simulink model "missile_Lin_model"  (R2022b)
settings: Solver=VariableStepAuto  StartTime=0.0  StopTime=10.0  RelTol=1e-3
InitFcn:
  | UAV_Data
  | Sim_Parameters
values from neighbouring files (symbols this model uses):
  D = 0.150    (= 0.15)    [UAV_Data.m]    (also in UAV_Data.mat)
  I_TENSOR = [ I_xx,  0.0,  0.0 ... (first row only)    [UAV_Data.m]    (also in UAV_Data.mat = [0.084375  0  0; 0  6.5869975  0; 0  0  6.5869975])
  Init_Euler = [ 0, 0.0, 0.0 ] *  UNIT_DEG2RAD    [Sim_Parameters.m]    (also in main_Assigment3.m = [ 0.0, 0.0, 0.0 ]')
  Init_Pos = [ 0.0, 0.0, -1000.0 ]    [Sim_Parameters.m]    (also in main_Assigment3.m = [ 0.0, 0.0, -1000 ]')
  Init_Rate = [ 0, 0.0, 0.0 ] * UNIT_DEG2RAD    [Sim_Parameters.m]    (also in main_Assigment3.m = [ 0.0, 0.0, 0.0 ]')
  Init_Vel = [ 238.0, 0.0, 0.0 ]    [Sim_Parameters.m]    (also in main_Assigment3.m = [ 238, 0, 0]')
  Mass = 30.0    (= 30)    [UAV_Data.m]    (also in UAV_Data.mat)
  S = dat.S    [Assigment3_work.m]    (also in Missile_EoM.m; UAV_Data.m = 0.0176714586764; UAV_Data.mat = 0.0176714586764; verify_coeff.m)
  Theta_dot_Trim = 0.0 * UNIT_DEG2RAD    [Trim_Main_missile.m]
  Turn_dot_Trim = 0.0 * UNIT_DEG2RAD    [Trim_Main_missile.m]
  UNIT_GRAV = 9.81    [Sim_Parameters.m]
  XCG = 0.809    [UAV_Data.m]    (also in UAV_Data.mat)
  XREF = 0.809    [UAV_Data.m]    (also in UAV_Data.mat)
libraries: shared6dofsys x2, aerolibtransform2 x1, sharedtransform x1, sharedutil x1, aerolibatmos2 x1, aerolibbdyn x1
settings Model: Creator=Komsun  LastModifiedBy=Komsun

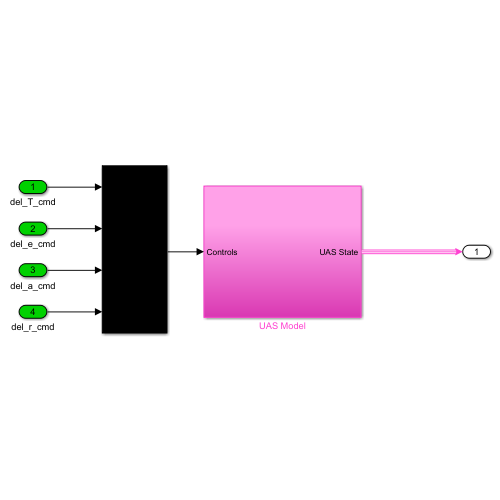
[thumbnail: Simulink's stored preview of the top-level diagram]
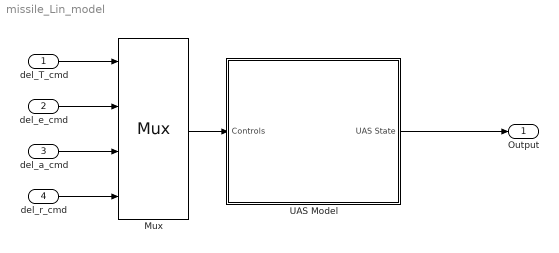
== system missile_Lin_model ==
  del_T_cmd : Inport
  del_e_cmd : Inport  Port=2
  del_a_cmd : Inport  Port=3
  del_r_cmd : Inport  Port=4
  Mux : Mux
  UAS Model : Subsystem
  Output : Outport
  wires:
  UAS Model/1(UAS State) -> Output/1
  del_T_cmd/1 -> Mux/1
  del_e_cmd/1 -> Mux/2
  del_r_cmd/1 -> Mux/4
  del_a_cmd/1 -> Mux/3
  Mux/1 -> UAS Model/1(Controls)

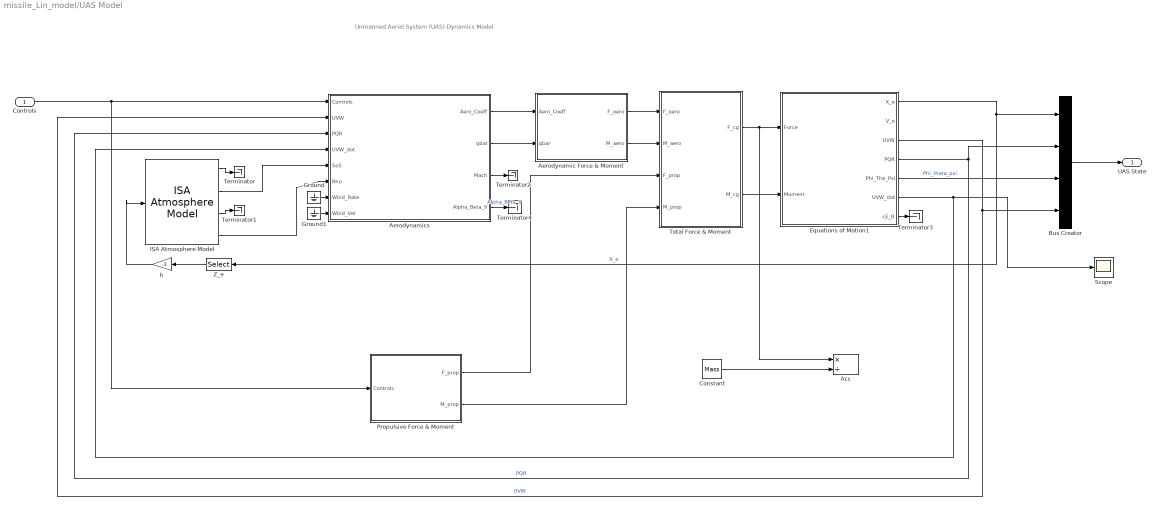
== system missile_Lin_model/UAS Model ==
  note: Unmanned Aerial System (UAS) Dynamics Model
  Controls : Inport
  Acc : Product  Inputs=*/  RndMeth=Zero
  Aerodynamic Force & Moment : Subsystem
  Aerodynamics : Subsystem
  Bus Creator : BusCreator  Inputs=4
  Constant : Constant  Value=Mass
  Equations of Motion1 : Subsystem
  Ground : Ground
  Ground1 : Ground
  ISA Atmosphere Model : aerolibatmos2/ISA Atmosphere Model  custom=off  g=9.80665  gamma=1.4  R=287.0531  L=0.0065  h_trop=11000  h_strat=20000  rho0=1.225  P0=101325  T0=288.15  h0=0
  Propulsive Force & Moment : Subsystem
  Scope : Scope
  Terminator{,1..4} (5 alike) : Terminator
  Total Force & Moment : Subsystem
  Z_e : Selector  InputPortWidth=3  IndexOptions=Index vector (dialog)  Indices=[3]  OutputSizes=1
  h : Gain  Gain=-1
  UAS State : Outport
  wires:
  ISA Atmosphere Model/2 -> Aerodynamics/5(SoS)
  ISA Atmosphere Model/4 -> Aerodynamics/6(Rho)
  ISA Atmosphere Model/1 -> Terminator/1
  ISA Atmosphere Model/3 -> Terminator1/1
  Aerodynamics/1(Aero_Coeff) -> Aerodynamic Force & Moment/1(Aero_Coeff)
  Aerodynamics/2(qbar) -> Aerodynamic Force & Moment/2(qbar)
  Aerodynamics/3(Mach) -> Terminator2/1
  Aerodynamic Force & Moment/1(F_aero) -> Total Force & Moment/1(F_aero)
  Aerodynamic Force & Moment/2(M_aero) -> Total Force & Moment/2(M_aero)
  Controls/1 -> Propulsive Force & Moment/1(Controls), Aerodynamics/1(Controls)
  Propulsive Force & Moment/1(F_prop) -> Total Force & Moment/3(F_prop)
  Propulsive Force & Moment/2(M_prop) -> Total Force & Moment/4(M_prop)
  Total Force & Moment/1(F_cg) -> Equations of Motion1/1(Force), Acc/1
  Total Force & Moment/2(M_cg) -> Equations of Motion1/2(Moment)
  Constant/1 -> Acc/2
  Bus Creator/1 -> UAS State/1
  Equations of Motion1/1(X_e) -> Bus Creator/1, Z_e/1  "X_e"
  Z_e/1 -> h/1
  h/1 -> ISA Atmosphere Model/1
  Equations of Motion1/3(UVW) -> Bus Creator/4, Aerodynamics/2(UVW)  "UVW"
  Equations of Motion1/6(UVW_dot) -> Scope/1, Aerodynamics/4("UVW_dot ")
  Equations of Motion1/4(PQR) -> Bus Creator/2, Aerodynamics/3(PQR)  "PQR"
  Equations of Motion1/5(Phi_The_Psi) -> Bus Creator/3  "Phi_theta_psi"
  Equations of Motion1/7(cE_B) -> Terminator3/1
  Ground/1 -> Aerodynamics/7(Wind_Rate)
  Ground1/1 -> Aerodynamics/8(Wind_Vel)
  Aerodynamics/4(Alpha_Beta_V) -> Terminator4/1  "Alpha_Beta_V"

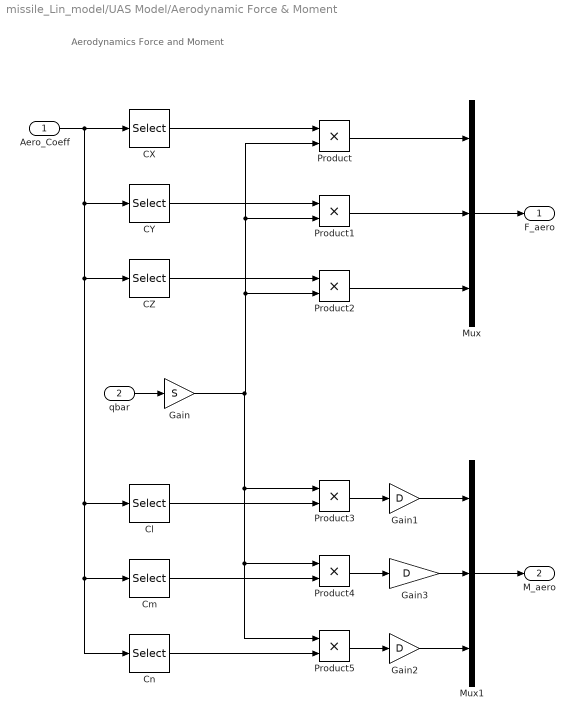
== system missile_Lin_model/UAS Model/Aerodynamic Force & Moment ==
  note: Aerodynamics Force and Moment
  Aero_Coeff : Inport
  qbar : Inport  Port=2
  CX : Selector  InputPortWidth=6  IndexOptions=Index vector (dialog)  Indices=[1]  OutputSizes=1
  CY : Selector  InputPortWidth=6  IndexOptions=Index vector (dialog)  Indices=[2]  OutputSizes=1
  CZ : Selector  InputPortWidth=6  IndexOptions=Index vector (dialog)  Indices=[3]  OutputSizes=1
  Cl : Selector  InputPortWidth=6  IndexOptions=Index vector (dialog)  Indices=[4]  OutputSizes=1
  Cm : Selector  InputPortWidth=6  IndexOptions=Index vector (dialog)  Indices=[5]  OutputSizes=1
  Cn : Selector  InputPortWidth=6  IndexOptions=Index vector (dialog)  Indices=[6]  OutputSizes=1
  Gain : Gain  Gain=S
  Gain1 : Gain  Gain=D
  Gain2 : Gain  Gain=D
  Gain3 : Gain  Gain=D
  Mux : Mux  Inputs=3
  Mux1 : Mux  Inputs=3
  Product{,1..5} (6 alike) : Product
  F_aero : Outport
  M_aero : Outport  Port=2
  wires:
  Aero_Coeff/1 -> Cl/1, Cn/1, Cm/1, CZ/1, CY/1, CX/1
  qbar/1 -> Gain/1
  CX/1 -> Product/1
  Gain/1 -> Product5/1, Product4/1, Product3/1, Product2/2, Product1/2, Product/2
  CY/1 -> Product1/1
  CZ/1 -> Product2/1
  Product/1 -> Mux/1
  Product1/1 -> Mux/2
  Product2/1 -> Mux/3
  Mux/1 -> F_aero/1
  Cl/1 -> Product3/2
  Cm/1 -> Product4/2
  Cn/1 -> Product5/2
  Product3/1 -> Gain1/1
  Product4/1 -> Gain3/1
  Product5/1 -> Gain2/1
  Mux1/1 -> M_aero/1
  Gain1/1 -> Mux1/1
  Gain2/1 -> Mux1/3
  Gain3/1 -> Mux1/2

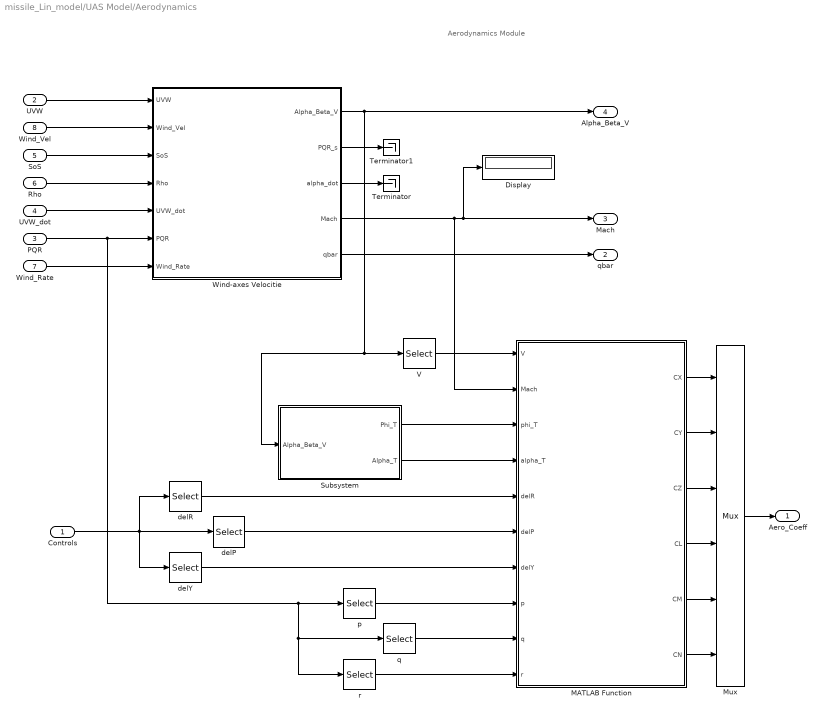
== system missile_Lin_model/UAS Model/Aerodynamics ==
  note: Aerodynamics Module
  Controls : Inport
  UVW : Inport  Port=2
  PQR : Inport  Port=3
  "UVW_dot " : Inport  Port=4
  SoS : Inport  Port=5
  Rho : Inport  Port=6
  Wind_Rate : Inport  Port=7
  Wind_Vel : Inport  Port=8
  Display : Display
  MATLAB Function : MATLAB Function  TreatAsAtomicUnit=on
  Mux : Mux  Inputs=6
  Subsystem : Subsystem
  Terminator : Terminator
  Terminator1 : Terminator
  V : Selector  InputPortWidth=3  IndexOptions=Index vector (dialog)  Indices=[3]  OutputSizes=1
  Wind-axes Velocitie : Subsystem
  delP : Selector  InputPortWidth=4  IndexOptions=Index vector (dialog)  Indices=[3]  OutputSizes=1
  delR : Selector  InputPortWidth=4  IndexOptions=Index vector (dialog)  Indices=[2]  OutputSizes=1
  delY : Selector  InputPortWidth=4  IndexOptions=Index vector (dialog)  Indices=[4]  OutputSizes=1
  p : Selector  InputPortWidth=3  IndexOptions=Index vector (dialog)  Indices=[1]  OutputSizes=1
  q : Selector  InputPortWidth=3  IndexOptions=Index vector (dialog)  Indices=[2]  OutputSizes=1
  r : Selector  InputPortWidth=3  IndexOptions=Index vector (dialog)  Indices=[3]  OutputSizes=1
  Aero_Coeff : Outport
  qbar : Outport  Port=2
  Mach : Outport  Port=3
  Alpha_Beta_V : Outport  Port=4
  wires:
  Wind-axes Velocitie/1(Alpha_Beta_V) -> Subsystem/1(Alpha_Beta_V), V/1, Alpha_Beta_V/1
  UVW/1 -> Wind-axes Velocitie/1(UVW)
  Mux/1 -> Aero_Coeff/1
  Wind-axes Velocitie/4(Mach) -> MATLAB Function/2(Mach), Mach/1, Display/1
  Wind-axes Velocitie/5(qbar) -> qbar/1
  Wind_Vel/1 -> Wind-axes Velocitie/2(Wind_Vel)
  SoS/1 -> Wind-axes Velocitie/3(SoS)
  Rho/1 -> Wind-axes Velocitie/4(Rho)
  "UVW_dot "/1 -> Wind-axes Velocitie/5(UVW_dot)
  PQR/1 -> r/1, q/1, p/1, Wind-axes Velocitie/6(PQR)
  Wind_Rate/1 -> Wind-axes Velocitie/7(Wind_Rate)
  MATLAB Function/1(CX) -> Mux/1
  MATLAB Function/2(CY) -> Mux/2
  MATLAB Function/3(CZ) -> Mux/3
  MATLAB Function/4(CL) -> Mux/4
  MATLAB Function/5(CM) -> Mux/5
  MATLAB Function/6(CN) -> Mux/6
  Wind-axes Velocitie/3(alpha_dot) -> Terminator/1
  Wind-axes Velocitie/2(PQR_s) -> Terminator1/1
  Subsystem/2(Alpha_T) -> MATLAB Function/4(alpha_T)
  V/1 -> MATLAB Function/1(V)
  Subsystem/1(Phi_T) -> MATLAB Function/3(phi_T)
  Controls/1 -> delY/1, delR/1, delP/1
  delR/1 -> MATLAB Function/5(delR)
  delP/1 -> MATLAB Function/6(delP)
  delY/1 -> MATLAB Function/7(delY)
  p/1 -> MATLAB Function/8(p)
  q/1 -> MATLAB Function/9(q)
  r/1 -> MATLAB Function/10(r)

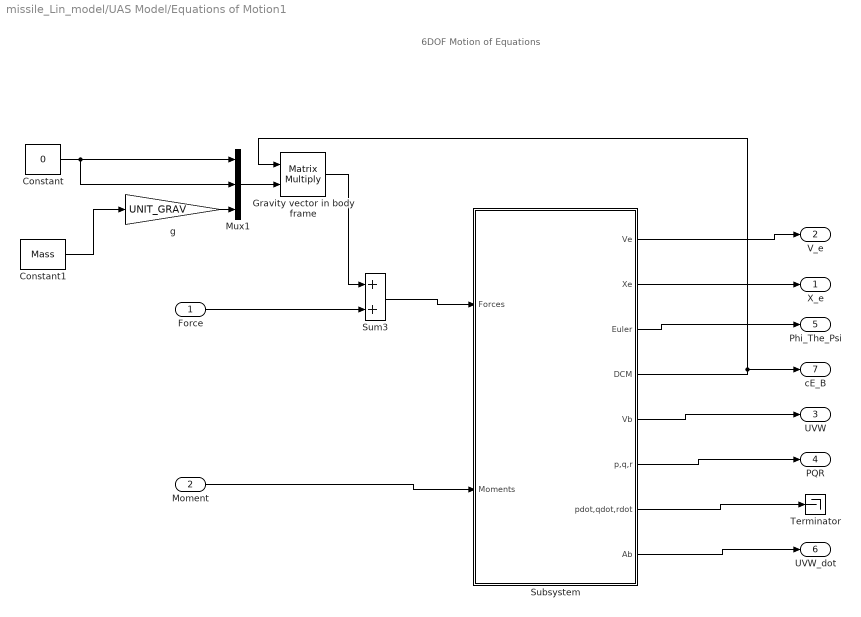
== system missile_Lin_model/UAS Model/Equations of Motion1 ==
  note: 6DOF Motion of Equations
  Force : Inport  PortDimensions=3
  Moment : Inport  Port=2  PortDimensions=3
  Constant : Constant  Value=0
  Constant1 : Constant  Value=Mass
  "Gravity vector in body frame " : Product  Multiplication=Matrix(*)  InputSameDT=on  SaturateOnIntegerOverflow=on  OutDataTypeStr=Inherit: Same as first input
  Mux1 : Mux  Inputs=3
  Subsystem : Subsystem
  Sum3 : Sum  InputSameDT=on  SaturateOnIntegerOverflow=on  OutDataTypeStr=Inherit: Same as first input
  Terminator : Terminator
  g : Gain  Gain=UNIT_GRAV
  X_e : Outport
  V_e : Outport  Port=2
  UVW : Outport  Port=3
  PQR : Outport  Port=4
  Phi_The_Psi : Outport  Port=5
  UVW_dot : Outport  Port=6
  cE_B : Outport  Port=7
  wires:
  Sum3/1 -> Subsystem/1(Forces)
  g/1 -> Mux1/3
  "Gravity vector in body frame "/1 -> Sum3/1
  Constant/1 -> Mux1/2, Mux1/1
  Mux1/1 -> "Gravity vector in body frame "/2
  Force/1 -> Sum3/2
  Moment/1 -> Subsystem/2(Moments)
  Constant1/1 -> g/1
  Subsystem/1(Ve) -> V_e/1
  Subsystem/3(Euler) -> Phi_The_Psi/1
  Subsystem/4(DCM) -> "Gravity vector in body frame "/1, cE_B/1
  Subsystem/5(Vb) -> UVW/1
  Subsystem/6(p,q,r) -> PQR/1
  Subsystem/7(pdot,qdot,rdot) -> Terminator/1
  Subsystem/8(Ab) -> UVW_dot/1
  Subsystem/2(Xe) -> X_e/1

== system missile_Lin_model/UAS Model/Propulsive Force & Moment ==
  note: Propulsive Force and Moment
  Controls : Inport
  Constant : Constant  Value=0
  Mux : Mux  Inputs=3
  Mux1 : Mux  Inputs=3
  Thrust : Selector  InputPortWidth=4  IndexOptions=Index vector (dialog)  Indices=[1]  OutputSizes=1
  F_prop : Outport
  M_prop : Outport  Port=2
  wires:
  Mux1/1 -> M_prop/1
  Constant/1 -> Mux/3, Mux1/3, Mux1/2, Mux1/1, Mux/2
  Controls/1 -> Thrust/1
  Thrust/1 -> Mux/1
  Mux/1 -> F_prop/1

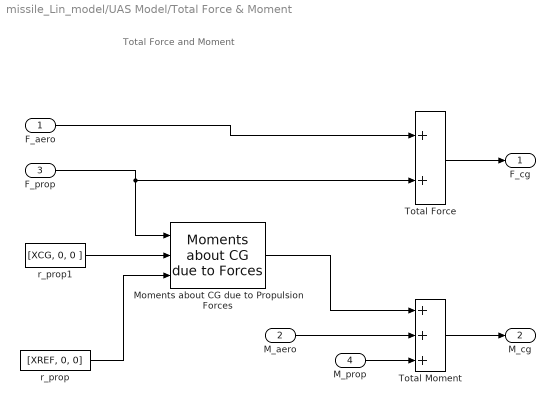
== system missile_Lin_model/UAS Model/Total Force & Moment ==
  note: Total Force and Moment
  F_aero : Inport  PortDimensions=3
  M_aero : Inport  Port=2  PortDimensions=3
  F_prop : Inport  Port=3  PortDimensions=3
  M_prop : Inport  Port=4  PortDimensions=3
  Moments about CG due to Propulsion Forces : aerolibbdyn/Moments about CG  due to Forces
  Total Force : Sum  InputSameDT=on  SaturateOnIntegerOverflow=on  OutDataTypeStr=Inherit: Same as first input
  Total Moment : Sum  Inputs=+++  InputSameDT=on  SaturateOnIntegerOverflow=on  OutDataTypeStr=Inherit: Same as first input
  r_prop : Constant  Value=[XREF, 0, 0]  OutDataTypeStr=double
  r_prop1 : Constant  Value=[XCG, 0, 0 ]  OutDataTypeStr=double
  F_cg : Outport
  M_cg : Outport  Port=2
  wires:
  M_aero/1 -> Total Moment/2
  Moments about CG due to Propulsion Forces/1 -> Total Moment/1
  Total Force/1 -> F_cg/1
  F_aero/1 -> Total Force/1
  F_prop/1 -> Moments about CG due to Propulsion Forces/1, Total Force/2
  M_prop/1 -> Total Moment/3
  Total Moment/1 -> M_cg/1
  r_prop/1 -> Moments about CG due to Propulsion Forces/3
  r_prop1/1 -> Moments about CG due to Propulsion Forces/2

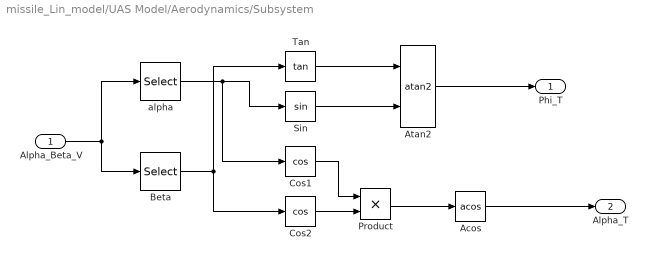
== system missile_Lin_model/UAS Model/Aerodynamics/Subsystem ==
  Alpha_Beta_V : Inport
  Acos : Trigonometry  Operator=acos
  Atan2 : Trigonometry  Operator=atan2
  Beta : Selector  InputPortWidth=3  IndexOptions=Index vector (dialog)  Indices=[2]  OutputSizes=1
  Cos1 : Trigonometry  Operator=cos
  Cos2 : Trigonometry  Operator=cos
  Product : Product
  Sin : Trigonometry
  Tan : Trigonometry  Operator=tan
  alpha : Selector  InputPortWidth=3  IndexOptions=Index vector (dialog)  Indices=[1]  OutputSizes=1
  Phi_T : Outport
  Alpha_T : Outport  Port=2
  wires:
  Alpha_Beta_V/1 -> alpha/1, Beta/1
  Beta/1 -> Tan/1, Cos2/1
  Tan/1 -> Atan2/1
  Sin/1 -> Atan2/2
  Atan2/1 -> Phi_T/1
  alpha/1 -> Cos1/1, Sin/1
  Cos1/1 -> Product/1
  Cos2/1 -> Product/2
  Product/1 -> Acos/1
  Acos/1 -> Alpha_T/1

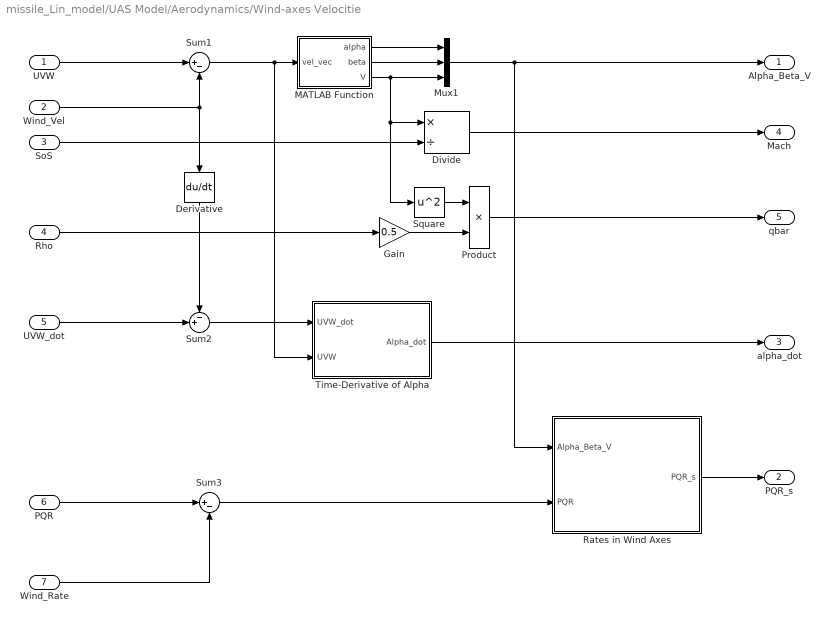
== system missile_Lin_model/UAS Model/Aerodynamics/Wind-axes Velocitie ==
  UVW : Inport
  Wind_Vel : Inport  Port=2
  SoS : Inport  Port=3
  Rho : Inport  Port=4
  UVW_dot : Inport  Port=5
  PQR : Inport  Port=6
  Wind_Rate : Inport  Port=7
  Derivative : Derivative
  Divide : Product  Inputs=*/
  Gain : Gain  Gain=0.5
  MATLAB Function : MATLAB Function  TreatAsAtomicUnit=on
  Mux1 : Mux  Inputs=3
  Product : Product
  Rates in Wind Axes : Subsystem
  Square : Math  Operator=square
  Sum1 : Sum  Inputs=|+-  InputSameDT=on  SaturateOnIntegerOverflow=on  OutDataTypeStr=Inherit: Same as first input
  Sum2 : Sum  Inputs=-+|  InputSameDT=on  SaturateOnIntegerOverflow=on  OutDataTypeStr=Inherit: Same as first input
  Sum3 : Sum  Inputs=|+-  InputSameDT=on  SaturateOnIntegerOverflow=on  OutDataTypeStr=Inherit: Same as first input
  Time-Derivative of Alpha : Subsystem
  Alpha_Beta_V : Outport
  PQR_s : Outport  Port=2
  alpha_dot : Outport  Port=3
  Mach : Outport  Port=4
  qbar : Outport  Port=5
  wires:
  Derivative/1 -> Sum2/1
  Sum2/1 -> Time-Derivative of Alpha/1(UVW_dot)
  UVW_dot/1 -> Sum2/2
  Time-Derivative of Alpha/1(Alpha_dot) -> alpha_dot/1
  Product/1 -> qbar/1
  Rho/1 -> Gain/1
  SoS/1 -> Divide/2
  Divide/1 -> Mach/1
  Wind_Vel/1 -> Sum1/2, Derivative/1
  UVW/1 -> Sum1/1
  Mux1/1 -> Rates in Wind Axes/1(Alpha_Beta_V), Alpha_Beta_V/1
  Sum1/1 -> Time-Derivative of Alpha/2(UVW), MATLAB Function/1(vel_vec)
  MATLAB Function/1(alpha) -> Mux1/1
  MATLAB Function/2(beta) -> Mux1/2
  MATLAB Function/3(V) -> Square/1, Divide/1, Mux1/3
  Rates in Wind Axes/1(PQR_s) -> PQR_s/1
  Sum3/1 -> Rates in Wind Axes/2(PQR)
  PQR/1 -> Sum3/1
  Wind_Rate/1 -> Sum3/2
  Square/1 -> Product/1
  Gain/1 -> Product/2

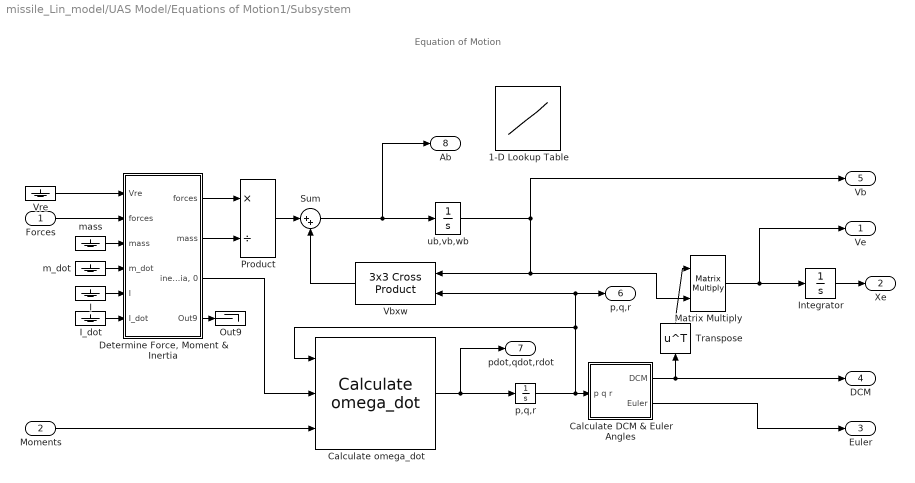
== system missile_Lin_model/UAS Model/Equations of Motion1/Subsystem ==
  note: Equation of Motion
  Forces : Inport  PortDimensions=3
  Moments : Inport  Port=2  PortDimensions=3
  1-D Lookup Table : Lookup_n-D  NumberOfTableDimensions=1  BreakpointsForDimension1=[-5:5]  Table=tanh([-5:5])  InternalRulePriority=Speed  RndMeth=Simplest
  Calculate DCM & Euler Angles : Subsystem
  Calculate omega_dot : shared6dofsys/Calculate omega_dot  aMode=aMode
  "Determine Force, Moment & Inertia" : Subsystem
  I : Ground
  I_dot : Ground
  Integrator : Integrator  InitialCondition=Init_Pos
  Matrix Multiply : Product  Multiplication=Matrix(*)
  Out9 : Terminator
  Product : Product  Inputs=*/  SaturateOnIntegerOverflow=on  OutDataTypeStr=Inherit: Same as first input
  Sum : Sum  Inputs=|++  SaturateOnIntegerOverflow=on
  Transpose : Math  Operator=transpose  SignedPower=on
  Vbxw : sharedutil/3x3 Cross Product  aMode=aMode
      settings: LibrarySourceBlock=aerolibutil/3x3 Cross Product
  Vre : Ground
  m_dot : Ground
  mass : Ground
  "p,q,r " : Integrator  InitialCondition=Init_Rate
  ub,vb,wb : Integrator  InitialCondition=Init_Vel
  Ve : Outport
  Xe : Outport  Port=2
  Euler : Outport  Port=3
  DCM : Outport  Port=4
  Vb : Outport  Port=5
  p,q,r : Outport  Port=6
  pdot,qdot,rdot : Outport  Port=7
  Ab : Outport  Port=8
  wires:
  Matrix Multiply/1 -> Integrator/1, Ve/1
  ub,vb,wb/1 -> Vb/1, Matrix Multiply/2, Vbxw/1
  Vre/1 -> "Determine Force, Moment & Inertia"/1(Vre)
  "Determine Force, Moment & Inertia"/1("forces ") -> Product/1
  I_dot/1 -> "Determine Force, Moment & Inertia"/6(I_dot)
  I/1 -> "Determine Force, Moment & Inertia"/5(I)
  Calculate omega_dot/1 -> "p,q,r "/1, pdot,qdot,rdot/1
  "Determine Force, Moment & Inertia"/4(Out9) -> Out9/1
  m_dot/1 -> "Determine Force, Moment & Inertia"/4(m_dot)
  mass/1 -> "Determine Force, Moment & Inertia"/3("mass ")
  Transpose/1 -> Matrix Multiply/1
  Calculate DCM & Euler Angles/1(DCM) -> Transpose/1, DCM/1
  Product/1 -> Sum/1
  Forces/1 -> "Determine Force, Moment & Inertia"/2(forces)
  Moments/1 -> Calculate omega_dot/3
  "p,q,r "/1 -> Calculate DCM & Euler Angles/1("p q r "), Vbxw/2, p,q,r/1, Calculate omega_dot/1
  Vbxw/1 -> Sum/2
  Calculate DCM & Euler Angles/2(Euler) -> Euler/1
  "Determine Force, Moment & Inertia"/2(mass) -> Product/2
  "Determine Force, Moment & Inertia"/3("inertia, 0") -> Calculate omega_dot/2
  Sum/1 -> Ab/1, ub,vb,wb/1
  Integrator/1 -> Xe/1

== system missile_Lin_model/UAS Model/Aerodynamics/Wind-axes Velocitie/Rates in Wind Axes ==
  note: Rates in Wind Axes
  Alpha_Beta_V : Inport
  PQR : Inport  Port=2
  Alpha : Selector  InputPortWidth=3  IndexOptions=Index vector (dialog)  Indices=[1]  OutputSizes=1
  Beta_Ref : Constant  Value=0
  Direction Cosine Matrix Body to Wind : aerolibtransform2/Direction Cosine Matrix Body to Wind
  Mux : Mux  Inputs=2
  transform to body axes : Product  Inputs=**  Multiplication=Matrix(*)  InputSameDT=on  SaturateOnIntegerOverflow=on  OutDataTypeStr=Inherit: Same as first input
  PQR_s : Outport
  wires:
  Alpha_Beta_V/1 -> Alpha/1
  Alpha/1 -> Mux/1
  Direction Cosine Matrix Body to Wind/1 -> transform to body axes/1  "cB_W"
  PQR/1 -> transform to body axes/2
  transform to body axes/1 -> PQR_s/1
  Mux/1 -> Direction Cosine Matrix Body to Wind/1
  Beta_Ref/1 -> Mux/2

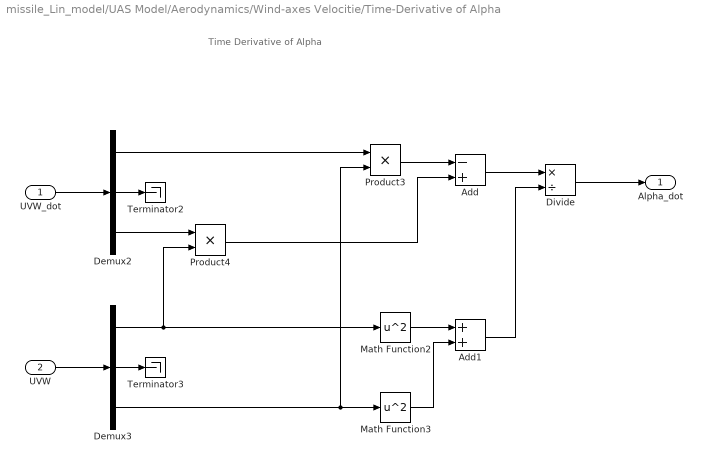
== system missile_Lin_model/UAS Model/Aerodynamics/Wind-axes Velocitie/Time-Derivative of Alpha ==
  note: Time Derivative of Alpha
  UVW_dot : Inport
  UVW : Inport  Port=2
  Add : Sum  Inputs=-+
  Add1 : Sum
  Demux2 : Demux  Outputs=3
  Demux3 : Demux  Outputs=3
  Divide : Product  Inputs=*/
  Math Function2 : Math  Operator=square  SignedPower=on
  Math Function3 : Math  Operator=square  SignedPower=on
  Product3 : Product
  Product4 : Product
  Terminator2 : Terminator
  Terminator3 : Terminator
  Alpha_dot : Outport
  wires:
  UVW_dot/1 -> Demux2/1
  Demux2/2 -> Terminator2/1
  Demux2/1 -> Product3/1
  UVW/1 -> Demux3/1
  Demux3/2 -> Terminator3/1
  Demux3/3 -> Math Function3/1, Product3/2
  Demux2/3 -> Product4/1
  Demux3/1 -> Math Function2/1, Product4/2
  Product4/1 -> Add/2
  Product3/1 -> Add/1
  Add/1 -> Divide/1
  Math Function2/1 -> Add1/1
  Math Function3/1 -> Add1/2
  Add1/1 -> Divide/2
  Divide/1 -> Alpha_dot/1

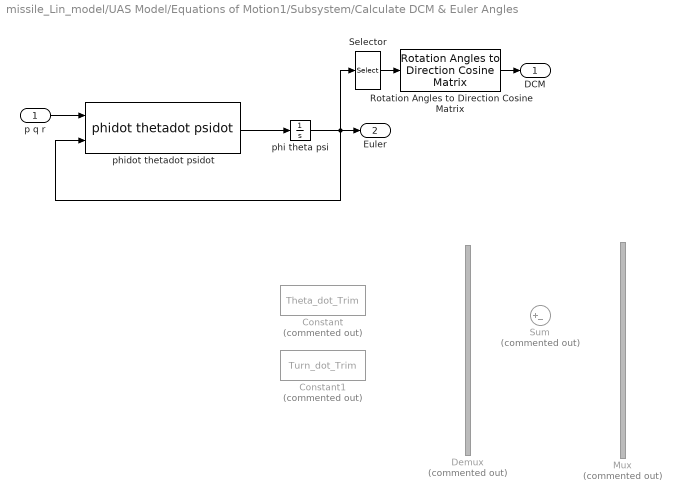
== system missile_Lin_model/UAS Model/Equations of Motion1/Subsystem/Calculate DCM & Euler Angles ==
  "p q r " : Inport
  Constant : Constant  Commented=on  Value=Theta_dot_Trim
  Constant1 : Constant  Commented=on  Value=Turn_dot_Trim
  Demux : Demux  Commented=on  Outputs=3
  Mux : Mux  Commented=on  Inputs=3
  Rotation Angles to Direction Cosine Matrix : sharedtransform/Rotation Angles to Direction Cosine Matrix  rotationOrder=ZYX  aMode=aMode
  Selector : Selector  InputPortWidth=3  IndexOptions=Index vector (dialog)  Indices=[3 2 1]  OutputSizes=1
  Sum : Sum  Commented=on  Inputs=|+-
  phi theta psi : Integrator  InitialCondition=Init_Euler
  phidot thetadot psidot : shared6dofsys/DCM & Euler Angles (Euler)/phidot thetadot psidot  SystemSampleTime=-1  VariantActivationTime=update diagram  Latency=0  AutoFrameSizeCalculation=off
  DCM : Outport
  Euler : Outport  Port=2
  wires:
  Selector/1 -> Rotation Angles to Direction Cosine Matrix/1
  phi theta psi/1 -> phidot thetadot psidot/2, Selector/1, Euler/1
  phidot thetadot psidot/1 -> phi theta psi/1
  "p q r "/1 -> phidot thetadot psidot/1
  Rotation Angles to Direction Cosine Matrix/1 -> DCM/1

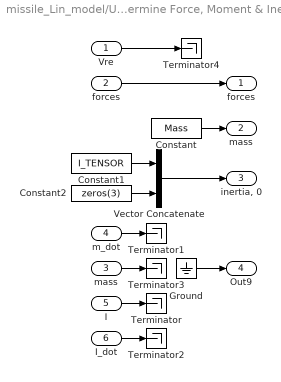
== system missile_Lin_model/UAS Model/Equations of Motion1/Subsystem/Determine Force, Moment & Inertia ==
  Vre : Inport
  forces : Inport  Port=2
  "mass " : Inport  Port=3
  m_dot : Inport  Port=4  OutDataTypeStr=double
  I : Inport  Port=5  OutDataTypeStr=double
  I_dot : Inport  Port=6  OutDataTypeStr=double
  Constant : Constant  Value=Mass  OutDataTypeStr=Inherit: Inherit via back propagation
  Constant1 : Constant  Value=I_TENSOR  OutDataTypeStr=Inherit: Inherit via back propagation
  Constant2 : Constant  Value=zeros(3)
  Ground : Ground
  Terminator{,1..4} (5 alike) : Terminator
  Vector Concatenate : Concatenate  Mode=Multidimensional array
  "forces " : Outport
  mass : Outport  Port=2
  "inertia, 0" : Outport  Port=3
  Out9 : Outport  Port=4
  wires:
  Vector Concatenate/1 -> "inertia, 0"/1
  Constant2/1 -> Vector Concatenate/2
  Constant1/1 -> Vector Concatenate/1
  Vre/1 -> Terminator4/1
  forces/1 -> "forces "/1
  "mass "/1 -> Terminator3/1
  I_dot/1 -> Terminator2/1
  m_dot/1 -> Terminator1/1
  I/1 -> Terminator/1
  Ground/1 -> Out9/1
  Constant/1 -> mass/1

== matlab function missile_Lin_model/UAS Model/Aerodynamics/Wind-axes Velocitie/MATLAB Function ==
  data: vel_vec input; alpha output; beta output; V output
function [alpha, beta, V] = calc_abv(vel_vec)

u = vel_vec(1);
v = vel_vec(2);
w = vel_vec(3);

V = norm([u v w]);          % [m/s] UAV total Speed
alpha = atan2(w,u);          % [rad] angle of attack
beta  = asin(v/V);          % [rad] sideslip angles

end

== matlab function missile_Lin_model/UAS Model/Aerodynamics/MATLAB Function ==
  data: V input; Mach input; CX output; phi_T input; alpha_T input; delR input; delP input; delY input; CY output; CZ output; CL output; CM output; CN output; p input; q input; r input
function [CX, CY, CZ, CL, CM, CN] = AeroCoef(V, Mach,phi_T, alpha_T, delR, delP, delY, p, q, r)

dat = load('UAV_Data.mat');
% dat.Tbl_ALPHAT = dat.Tbl_ALPHAT * pi/180;    % convert to rad
% alpha_T = alpha_T *180/pi;            % convert to degree

del_eff = (abs(delP) + abs(delY))/2;


B2A = rot1(-phi_T);                            % Body-to-Aeroballistics

delARPY = B2A *[delR; delP; delY];
delR_A = delARPY(1);
delP_A = delARPY(2);
delY_A = delARPY(3);

pqrA = B2A * [p; q; r];
pA = pqrA(1);
qA = pqrA(2);
rA = pqrA(3);

method = 'spline'; % 'spline', 'nearest'

CX_a = interp1(dat.Tbl_MACH, dat.Tbl_CX_0, Mach, method) + interp1(dat.Tbl_MACH, dat.Tbl_CX_ALPHAT, Mach, method)*alpha_T...
     + interp1(dat.Tbl_MACH, dat.Tbl_CX_DEL_EFF, Mach, method)*(del_eff)^2;

CY_a = interp2(dat.Tbl_ALPHAT, dat.Tbl_MACH, dat.Tbl_CY_PHIT, alpha_T*180/pi, Mach, method)*sin(4*phi_T)...
     + interp1(dat.Tbl_MACH, dat.Tbl_CY_DEL_Y, Mach, method)*delY_A;

CZ_a = interp2(dat.Tbl_ALPHAT, dat.Tbl_MACH, dat.Tbl_CZ_0, alpha_T*180/pi, Mach, method)...
     + interp2(dat.Tbl_ALPHAT, dat.Tbl_MACH, dat.Tbl_CZ_PHIT, alpha_T*180/pi, Mach, method)*(sin(2*phi_T))^2 ...
     + interp1(dat.Tbl_MACH, dat.Tbl_CZ_DEL_P, Mach, method)*delP_A;

CL_a = interp1(dat.Tbl_MACH, dat.Tbl_CL_ALPHAT, Mach, method)*(alpha_T^2)*sin(4*phi_T) ...
     + interp1(dat.Tbl_MACH, dat.Tbl_CL_P, Mach, method)*(dat.D/(2*V))*pA ...
     + interp1(dat.Tbl_MACH, dat.Tbl_CL_DEL_R, Mach, method)*delR_A;

CM_a = interp2(dat.Tbl_ALPHAT, dat.Tbl_MACH, dat.Tbl_CM_0, alpha_T*180/pi, Mach, method) ...
     + interp2(dat.Tbl_ALPHAT, dat.Tbl_MACH, dat.Tbl_CM_PHIT, alpha_T*180/pi, Mach, method)*(sin(2*phi_T))^2 ...
     + interp1(dat.Tbl_MACH, dat.Tbl_CM_Q, Mach, method)*(dat.D/(2*V))*qA ...
     + interp1(dat.Tbl_MACH, dat.Tbl_CM_DEL_P, Mach, method)*delP_A ...
     - CZ_a*(dat.XCG - dat.XREF)/dat.D;

CN_a = interp2(dat.Tbl_ALPHAT, dat.Tbl_MACH, dat.Tbl_CN_PHIT, alpha_T*180/pi, Mach, method)*sin(4*phi_T)...
     + interp1(dat.Tbl_MACH, dat.Tbl_CN_R, Mach, method)*(dat.D/(2*V))*rA ...
     + interp1(dat.Tbl_MACH, dat.Tbl_CN_DEL_Y, Mach, method)*delY_A ...
     + CY_a*(dat.XCG - dat.XREF)/dat.D;

%% Aerodynamics Coefficients in body coordinate
CXYZ = B2A.' * [CX_a; CY_a; CZ_a];
CX = CXYZ(1);
CY = CXYZ(2);
CZ = CXYZ(3);

CLMN = B2A.' * [CL_a; CM_a; CN_a];
CL = CLMN(1);
CM = CLMN(2);
CN = CLMN(3);

function out = rot1(x)
    out = [1 0 0; 0 cos(x) sin(x); 0 -sin(x) cos(x)];
end

end
